simulink model "Reforce_Experiment_FCS"  (R2021a)
settings: Solver=FixedStepDiscrete  StartTime=0.0  StopTime=Inf  FixedStep=Ts  RelTol=1e-3
PostLoadFcn:
  | , if any(exist('dsrtsu_mdlpostloadfcn', 'file') ~= 0), dsrtsu_mdlpostloadfcn('Execute', bdroot); end,
InitFcn:
  | , if any(exist('rtifpga_mdlclblib', 'file') ~= 0), rtifpga_mdlclblib('Init', bdroot); end,
model workspace (MAT data in the model file):
  FPGA_Control_Scheme_1_Buffer_1_1_1_write : Simulink.Signal (value not decoded)
  FPGA_Control_Scheme_1_Buffer_2_1_1_write : Simulink.Signal (value not decoded)
  FPGA_Control_Scheme_1_Register_1_1_1_write : Simulink.Signal (value not decoded)
  FPGA_Control_Scheme_1_Register_2_1_1_write : Simulink.Signal (value not decoded)
values from neighbouring files (symbols this model uses):
  abc2alphabeta0 = [      2/3      -1/3       -1/3 ... (first row only)    [Reforce_Init.m]
  alphabeta02abc = [  1          0 1/sqrt(2) ... (first row only)    [Reforce_Init.m]
  torque_ref_sample_lower = -torque_ref_sample_upper    (= -6.5)    [Reforce_Init.m]
  torque_ref_sample_upper = 6.5    [Reforce_Init.m]
  Ts = 50e-6    (= 5e-05)    [Reforce_Init.m]
undefined symbols (not defined in the file or in its folder): controller, gcbh, init_layer_0, init_layer_1, init_layer_2, init_layer_3, init_layer_4, init_layer_5, init_layer_6, init_layer_7, init_layer_8, init_layer_9, inverter, load, motor, PLL, rtimp_mpsetup_gui, sensor
libraries: simulink x14, rtiproclib x13, rti1202lib_adc_class1 x8, rti1202lib_dio_class1 x4, dspfdesign x4, rtiemclib x2, rti1202lib_dac_class1 x1, embmathops x1, rti1202lib_base x1, rtitasklib x1, dsextras x1, simulink_extras x1
(part 5 of 5)

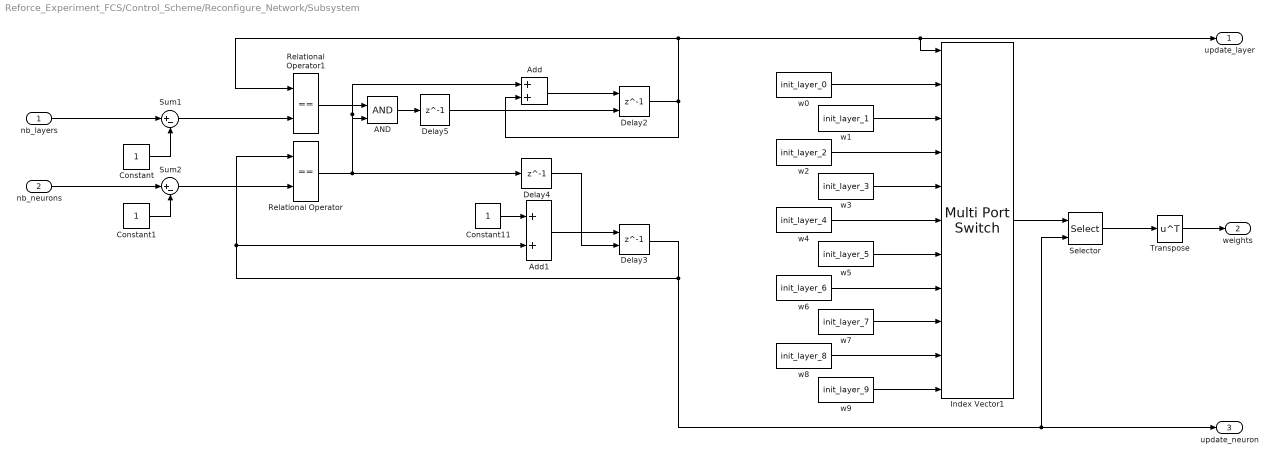
== system Reforce_Experiment_FCS/Control_Scheme/Reconfigure_Network/Subsystem ==
  nb_layers : Inport
  nb_neurons : Inport  Port=2
  AND : Logic  IconShape=distinctive  AllPortsSameDT=off  OutDataTypeStr=boolean
  Add : Sum
  Add1 : Sum
  Constant : Constant
  Constant1 : Constant
  Constant11 : Constant
  Delay2 : Delay  DelayLength=1  ExternalReset=Rising
      settings: InputPortMap=u0,r5
  Delay3 : Delay  DelayLength=1  ExternalReset=Level hold
      settings: InputPortMap=u0,r5
  Delay4 : Delay  DelayLength=1
  Delay5 : Delay  DelayLength=1
  Index Vector1 : MultiPortSwitch  DataPortOrder=Zero-based contiguous  Inputs=10  zeroidx=on
  Relational Operator : RelationalOperator  Operator===  OutDataTypeStr=boolean  RndMeth=Simplest
  Relational Operator1 : RelationalOperator  Operator===  OutDataTypeStr=boolean  RndMeth=Simplest
  Selector : Selector  NumberOfDimensions=2  IndexMode=Zero-based  InputPortWidth=2  IndexOptions=Index vector (port),Select all  Indices=[1 3],1  OutputSizes=1,1
  Sum1 : Sum  Inputs=|+-
  Sum2 : Sum  Inputs=|+-
  Transpose : Math  Operator=transpose  SaturateOnIntegerOverflow=on
  w0 : Constant  Value=init_layer_0
  w1 : Constant  Value=init_layer_1
  w2 : Constant  Value=init_layer_2
  w3 : Constant  Value=init_layer_3
  w4 : Constant  Value=init_layer_4
  w5 : Constant  Value=init_layer_5
  w6 : Constant  Value=init_layer_6
  w7 : Constant  Value=init_layer_7
  w8 : Constant  Value=init_layer_8
  w9 : Constant  Value=init_layer_9
  update_layer : Outport
  weights : Outport  Port=2
  update_neuron : Outport  Port=3
  wires:
  Delay3/1 -> Add1/2, Relational Operator/1, update_neuron/1, Selector/2
  Relational Operator/1 -> AND/2, Add/1, Delay4/1
  Add1/1 -> Delay3/1
  AND/1 -> Delay5/1
  Selector/1 -> Transpose/1
  Index Vector1/1 -> Selector/1
  Delay5/1 -> Delay2/2
  Delay2/1 -> Relational Operator1/1, update_layer/1, Index Vector1/1, Add/2
  Sum1/1 -> Relational Operator1/2
  Constant/1 -> Sum1/2
  Delay4/1 -> Delay3/2
  Add/1 -> Delay2/1
  Constant11/1 -> Add1/1
  nb_neurons/1 -> Sum2/1
  Relational Operator1/1 -> AND/1
  Sum2/1 -> Relational Operator/2
  Constant1/1 -> Sum2/2
  Transpose/1 -> weights/1
  nb_layers/1 -> Sum1/1
  w0/1 -> Index Vector1/2
  w1/1 -> Index Vector1/3
  w2/1 -> Index Vector1/4
  w3/1 -> Index Vector1/5
  w4/1 -> Index Vector1/6
  w5/1 -> Index Vector1/7
  w6/1 -> Index Vector1/8
  w7/1 -> Index Vector1/9
  w8/1 -> Index Vector1/10
  w9/1 -> Index Vector1/11

== system Reforce_Experiment_FCS/Measurement/PLL/PLL ==
  note: %% PLL
      | PLL.fn  =  50;           % [Hz] closed-loop nominal frequency of PLL
      | PLL.d   =  1;            % [] closed-loop damping factor of PLL
      | PLL.Ki_Ta = (2*pi*PLL.fn)^2;    % [1/s^2] integral gain of PLL controller
      | PLL.Kp = 2*PLL.d*2*pi*PLL.fn;   % [1/s] proportional gain of PLL controller
  note: PLL advanced entfernt
  Ts : Inport
  phi_el_cs : Inport  Port=2
  Integrator : Subsystem
  Memory : Memory  InitialCondition=[1 0]  InheritSampleTime=on  LinearizeAsDelay=on
  PI-Regler : Subsystem
  phase discriminator : Subsystem
  rad2cs : Subsystem
  Omega_el : Outport
  wires:
  Ts/1 -> PI-Regler/1(Ts), Integrator/1(Ts [s])
  Memory/1 -> phase discriminator/2(phi_e[cs])  "phi [cs]"
  rad2cs/1(phi_p[cs]) -> Memory/1  "phi_p [cs]"
  phase discriminator/1(dphi) -> PI-Regler/2(dphi)
  Integrator/1(phi [rad]) -> rad2cs/1(phi)
  PI-Regler/2(omega (KP)) -> Integrator/2(omega [rad/s])
  PI-Regler/1(omega) -> Omega_el/1  "sig_omega"
  phi_el_cs/1 -> phase discriminator/1(phi_x[cs])

== system Reforce_Experiment_FCS/Measurement/PLL/angle modulo ==
  angle_rad : Inport
  Complex to Magnitude-Angle : ComplexToMagnitudeAngle  Output=Angle
  Magnitude-Angle to Complex : MagnitudeAngleToComplex  Input=Angle  ConstantPart=1
  "angle_[-pi, pi]" : Outport
  wires:
  Magnitude-Angle to Complex/1 -> Complex to Magnitude-Angle/1
  angle_rad/1 -> Magnitude-Angle to Complex/1
  Complex to Magnitude-Angle/1 -> "angle_[-pi, pi]"/1

== system Reforce_Experiment_FCS/Measurement/abc2dq/alphabeta02dq ==
  alphabeta0 : Inport
  epsilon : Inport  Port=2
  Cos : Trigonometry  Operator=cos  NumberOfDataPoints=64
  Demux : Demux  Outputs=3
  Gain1 : Gain  Gain=-1
  Gain2 : Gain  Gain=-1
  Mux : Mux  Inputs=2
  Product{,1..3} (4 alike) : Product
  Sin : Trigonometry  NumberOfDataPoints=64
  Sum : Sum  Inputs=|++
  Sum1 : Sum  Inputs=|++
  Terminator : Terminator
  dq : Outport
  wires:
  epsilon/1 -> Gain2/1
  alphabeta0/1 -> Demux/1
  Demux/3 -> Terminator/1
  Sum/1 -> Mux/1
  Sum1/1 -> Mux/2
  Mux/1 -> dq/1
  Demux/1 -> Product1/1, Product2/1
  Cos/1 -> Product1/2, Product3/2
  Product1/1 -> Sum/1
  Demux/2 -> Product3/1, Product/1
  Gain1/1 -> Product/2
  Product/1 -> Sum/2
  Product2/1 -> Sum1/1
  Sin/1 -> Gain1/1, Product2/2
  Product3/1 -> Sum1/2
  Gain2/1 -> Sin/1, Cos/1

== system Reforce_Experiment_FCS/RTI Data/RTI Data Store/RTI Data Store ==
  RTI Data Store : Subsystem  mask(RTI_DATA_STORE){}
      mask help:
      | RTI Data Store Block. This block is used by RTI to store internal model dependent data. Deleting this block will result in data loss.
      |
      | NEVER DELETE, COPY, OR MODIFY THIS BLOCK!
      mask Help:
      | RTI Data Store Block. This block is used by RTI to store internal model dependent data. Deleting this block will result in data loss.
      | 
      | NEVER DELETE, COPY, OR MODIFY THIS BLOCK!
      mask Display: text(0.5, 0.5, ' ', 'HorizontalAlignment', 'center');

== system Reforce_Experiment_FCS/Control_Scheme/DQ_DTC/Action_Processing/argmax ==
  Q_values : Inport
  Add : Sum  Inputs=+-
  Compare To Zero : simulink/Logic and Bit Operations/Compare To Zero  relop===  OutDataTypeStr=boolean
  Find Nonzero Elements : Find  NumberOfInputDimensions=3  IndexMode=Zero-based
  Max : MinMax  Function=max
  Min : MinMax
  Rate Transition : RateTransition  Commented=on
  argmax_Q : Outport
  wires:
  Q_values/1 -> Add/1, Max/1
  Max/1 -> Add/2
  Add/1 -> Compare To Zero/1
  Find Nonzero Elements/1 -> Min/1
  Min/1 -> argmax_Q/1
  Compare To Zero/1 -> Find Nonzero Elements/1

== system Reforce_Experiment_FCS/Control_Scheme/DQ_DTC/Featurizer/DC_link_scaling ==
  u_DC : Inport
  Add : Sum  Inputs=+-
  Add1 : Sum  Inputs=-+
  Add2 : Sum  Inputs=+-
  Constant : Constant  Value=controller.DQDTC.u_DC_max
  Constant1 : Constant  Value=controller.DQDTC.u_DC_min
  Constant2 : Constant
  Divide : Product  Inputs=*/
  Gain : Gain  Gain=2
  u_DC_norm : Outport
  wires:
  u_DC/1 -> Add/1
  Constant1/1 -> Add/2, Add1/1
  Add/1 -> Divide/1
  Constant/1 -> Add1/2
  Add1/1 -> Divide/2
  Divide/1 -> Gain/1
  Constant2/1 -> Add2/2
  Add2/1 -> u_DC_norm/1
  Gain/1 -> Add2/1

== system Reforce_Experiment_FCS/Control_Scheme/DQ_DTC/Featurizer/stator_current_scaling ==
  i_dq_norm : Inport
  Constant : Constant
  Demux : Demux  Outputs=2
  Gain1 : Gain  Gain=2
  Sqrt : Sqrt  SaturateOnIntegerOverflow=on
  Square : Math  Operator=square  SaturateOnIntegerOverflow=on
  Square1 : Math  Operator=square  SaturateOnIntegerOverflow=on
  Sum : Sum  Inputs=|++
  Sum1 : Sum  Inputs=|+-
  i_s_norm : Outport
  wires:
  Constant/1 -> Sum1/2
  Gain1/1 -> Sum1/1
  Square/1 -> Sum/1
  Sqrt/1 -> Gain1/1
  i_dq_norm/1 -> Demux/1
  Demux/2 -> Square1/1
  Sum/1 -> Sqrt/1
  Demux/1 -> Square/1
  Square1/1 -> Sum/2
  Sum1/1 -> i_s_norm/1

== system Reforce_Experiment_FCS/Control_Scheme/DQ_DTC/Identification_and_Safeguard/A_d_static ==
  w_me : Inport
  Constant : Constant  Value=-1/motor.param.tau_d
  Constant1 : Constant  Value=-1/motor.param.tau_q
  Constant2 : Constant  Value=eye(2)
  Gain : Gain  Gain=-motor.param.L_d / motor.param.L_q
  Gain1 : Gain  Gain=motor.param.L_q / motor.param.L_d
  Gain2 : Gain  Gain=motor.param.p
  Gain3 : Gain  Gain=Ts
  Mux : Mux
  Plus : Sum
  Reshape1 : Reshape  OutputDimensionality=Customize  OutputDimensions=[2,2]
  A_d : Outport
  wires:
  Mux/1 -> Reshape1/1
  Constant/1 -> Mux/1
  Constant1/1 -> Mux/4
  Gain/1 -> Mux/2
  w_me/1 -> Gain2/1
  Gain2/1 -> Gain1/1, Gain/1
  Gain1/1 -> Mux/3
  Reshape1/1 -> Gain3/1
  Gain3/1 -> Plus/2
  Constant2/1 -> Plus/1
  Plus/1 -> A_d/1

== system Reforce_Experiment_FCS/Control_Scheme/DQ_DTC/Identification_and_Safeguard/Brosch RLS ==
  reset : Inport
  i_dq : Inport  Port=2
  u_dq : Inport  Port=3
  Routing : Subsystem
  i_d_RLS : Subsystem
  lambda : Constant  Value=controller.RLS.lambda
  A : Outport
  B : Outport  Port=2
  E : Outport  Port=3
  wires:
  Routing/3(E) -> E/1
  u_dq/1 -> i_d_RLS/3(u_dq)
  i_dq/1 -> i_d_RLS/2(i_dq)
  Routing/2(B) -> B/1
  i_d_RLS/1(theta_d_k) -> Routing/1(theta_d)
  Routing/1(A) -> A/1
  lambda/1 -> i_d_RLS/4(lambda)
  reset/1 -> i_d_RLS/1(reset)
  i_d_RLS/2(theta_q_k) -> Routing/2(theta_q)

== system Reforce_Experiment_FCS/Control_Scheme/DQ_DTC/Identification_and_Safeguard/DeadTimeCompensationPredictor ==
  A : Inport
  B : Inport  Port=2
  E : Inport  Port=3
  i_dq : Inport  Port=4
  u_dq : Inport  Port=5
  Add : Sum  Inputs=3
  Matrix Multiply : Product  Multiplication=Matrix(*)
  Matrix Multiply1 : Product  Multiplication=Matrix(*)
  i_dq[k+1] : Outport
  wires:
  i_dq/1 -> Matrix Multiply/2
  Add/1 -> i_dq[k+1]/1
  B/1 -> Matrix Multiply1/1
  Matrix Multiply/1 -> Add/1
  A/1 -> Matrix Multiply/1
  u_dq/1 -> Matrix Multiply1/2
  Matrix Multiply1/1 -> Add/2
  E/1 -> Add/3

== system Reforce_Experiment_FCS/Control_Scheme/DQ_DTC/Identification_and_Safeguard/E_d_static ==
  w_me : Inport
  Constant : Constant  Value=0
  Gain : Gain  Gain=-motor.param.p*motor.param.psi_p/motor.param.L_q
  Gain1 : Gain  Gain=Ts
  Mux : Mux  Inputs=2
  E_d : Outport
  wires:
  Mux/1 -> E_d/1
  Constant/1 -> Mux/1
  w_me/1 -> Gain/1
  Gain/1 -> Gain1/1
  Gain1/1 -> Mux/2

== system Reforce_Experiment_FCS/Control_Scheme/DQ_DTC/Identification_and_Safeguard/Horizon1Predictor ==
  A : Inport
  B : Inport  Port=2
  E : Inport  Port=3
  lastControlSignal : Inport  Port=4
  u_DC : Inport  Port=5
  i_dq[k+1] : Inport  Port=6
  i_abc[k+1] : Inport  Port=7
  epsilon : Inport  Port=8
  T_interlock : Inport  Port=9
  i_threshold : Inport  Port=10
  Constant : Constant  Value=inverter.mapping
  Constant1 : Constant  Value=eye(2)
  Constant3 : Constant  Value=[0 0]
  For Each Subsystem : Subsystem  TreatAsAtomicUnit=on
  Matrix Multiply : Product  Multiplication=Matrix(*)
  Matrix Multiply2 : Product  Inputs=/  Multiplication=Matrix(*)
  Plus : Sum
  Plus1 : Sum  Inputs=+-
  all_i_dq[k+2] : Outport
  all_u_EMF[k+2] : Outport  Port=2
  wires:
  E/1 -> Plus/1, For Each Subsystem/1(E)
  A/1 -> Matrix Multiply/1, Plus1/2
  Matrix Multiply/1 -> Plus/2
  Constant/1 -> For Each Subsystem/6(nextControlSignal)
  Constant1/1 -> Plus1/1
  i_threshold/1 -> For Each Subsystem/12(i_threshold)
  T_interlock/1 -> For Each Subsystem/11(T_interlock)
  i_abc[k+1]/1 -> For Each Subsystem/9(i_abc)
  u_DC/1 -> For Each Subsystem/8(u_DC)
  Matrix Multiply2/1 -> For Each Subsystem/5(B_inv)
  B/1 -> Matrix Multiply2/1, For Each Subsystem/4(B)
  Plus1/1 -> For Each Subsystem/2(I_minus_A)
  Plus/1 -> For Each Subsystem/3(Ai_plus_E)
  For Each Subsystem/2(u_dq[k+2]) -> all_u_EMF[k+2]/1
  For Each Subsystem/1(i_dq[k+2]) -> all_i_dq[k+2]/1
  lastControlSignal/1 -> For Each Subsystem/7(lastControlSignal)
  Constant3/1 -> Matrix Multiply/2
  epsilon/1 -> For Each Subsystem/10(epsilon)

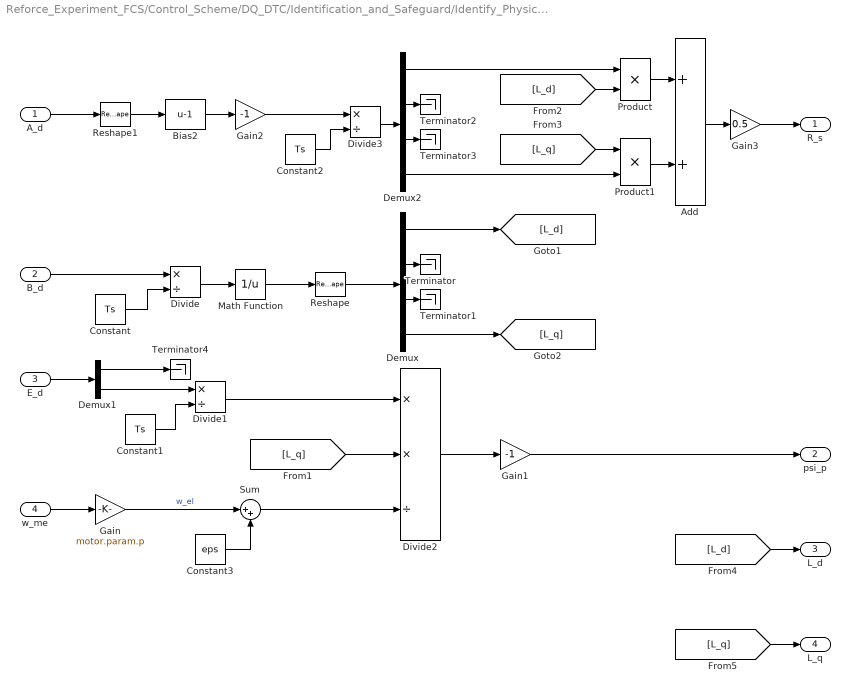
== system Reforce_Experiment_FCS/Control_Scheme/DQ_DTC/Identification_and_Safeguard/Identify_Physical_Parameters ==
  A_d : Inport
  B_d : Inport  Port=2
  E_d : Inport  Port=3
  w_me : Inport  Port=4
  Add : Sum
  Bias2 : Bias  Bias=-1
  Constant : Constant  Value=Ts
  Constant1 : Constant  Value=Ts
  Constant2 : Constant  Value=Ts
  Constant3 : Constant  Value=eps
  Demux : Demux
  Demux1 : Demux  Outputs=2
  Demux2 : Demux
  Divide : Product  Inputs=*/
  Divide1 : Product  Inputs=*/
  Divide2 : Product  Inputs=**/
  Divide3 : Product  Inputs=*/
  Gain : Gain  Gain=motor.param.p
  Gain1 : Gain  Gain=-1
  Gain2 : Gain  Gain=-1
  Gain3 : Gain  Gain=0.5
  Math Function : Math  Operator=reciprocal  SaturateOnIntegerOverflow=on
  Product : Product
  Product1 : Product
  Reshape : Reshape
  Reshape1 : Reshape
  Sum : Sum  Inputs=|++
  Terminator{,1..4} (5 alike) : Terminator
  R_s : Outport
  psi_p : Outport  Port=2
  L_d : Outport  Port=3
  L_q : Outport  Port=4
  wires:
  B_d/1 -> Divide/1
  Constant/1 -> Divide/2
  w_me/1 -> Gain/1
  Constant1/1 -> Divide1/2
  Divide1/1 -> Divide2/1
  Demux/1 -> [L_d]
  Reshape/1 -> Demux/1
  Demux/4 -> [L_q]
  Math Function/1 -> Reshape/1
  Demux/2 -> Terminator/1
  Demux/3 -> Terminator1/1
  Divide/1 -> Math Function/1
  [L_q] -> Divide2/2
  Divide2/1 -> Gain1/1
  Gain1/1 -> psi_p/1
  Reshape1/1 -> Bias2/1
  Demux2/3 -> Terminator3/1
  Demux2/2 -> Terminator2/1
  Bias2/1 -> Gain2/1
  A_d/1 -> Reshape1/1
  Constant2/1 -> Divide3/2
  Divide3/1 -> Demux2/1
  Gain2/1 -> Divide3/1
  Product/1 -> Add/1
  Product1/1 -> Add/2
  Add/1 -> Gain3/1
  Gain3/1 -> R_s/1
  Demux2/1 -> Product/1
  Demux2/4 -> Product1/2
  [L_q] -> Product1/1
  [L_d] -> Product/2
  [L_q] -> L_q/1
  [L_d] -> L_d/1
  Gain/1 -> Sum/1  "w_el"
  Sum/1 -> Divide2/3
  Constant3/1 -> Sum/2
  E_d/1 -> Demux1/1
  Demux1/2 -> Divide1/1
  Demux1/1 -> Terminator4/1

== system Reforce_Experiment_FCS/Control_Scheme/DQ_DTC/Identification_and_Safeguard/Safeguard ==
  i_dq : Inport
  u_dq : Inport  Port=2
  u_DC : Inport  Port=3
  Constant : Constant  Value=1:16
  Constant8 : Constant  Value=0:7
  For Each Subsystem : Subsystem  TreatAsAtomicUnit=on
  a_allowed : Outport
  all_i_s_feat : Outport  Port=2
  wires:
  u_dq/1 -> For Each Subsystem/2(u_dq)
  u_DC/1 -> For Each Subsystem/3(u_DC)
  For Each Subsystem/1(violation) -> a_allowed/1
  Constant8/1 -> For Each Subsystem/4(switch_state_index)
  For Each Subsystem/2(i_s_norm) -> all_i_s_feat/1
  Constant/1 -> For Each Subsystem/1(i_dq)

== system Reforce_Experiment_FCS/Control_Scheme/DQ_DTC/Identification_and_Safeguard/dq2abc ==
  dq : Inport
  epsilon : Inport  Port=2
  Gain1 : Gain  Gain=alphabeta02abc  Multiplication=Matrix(K*u)
  alphabeta02dq : Subsystem
  abc : Outport
  wires:
  epsilon/1 -> alphabeta02dq/2(epsilon)
  alphabeta02dq/1(alphabeta0) -> Gain1/1
  Gain1/1 -> abc/1
  dq/1 -> alphabeta02dq/1(dq)

== system Reforce_Experiment_FCS/Control_Scheme/DQ_DTC/Reward function/Zone A ==
  i_s : Inport
  Action Port : ActionPort  ActionPortLabel=else
  Add : Sum  Inputs=+-
  Constant : Constant
  Constant2 : Constant  Value=(controller.DQDTC.reward_interval)/2
  Constant3 : Constant  Value=0
  Gain1 : Gain  Gain=controller.DQDTC.reward_interval / 2
  Sum : Sum  Inputs=|++
  reward : Outport
  done : Outport  Port=2
  wires:
  Constant/1 -> Add/1
  i_s/1 -> Add/2
  Add/1 -> Gain1/1
  Gain1/1 -> Sum/1
  Sum/1 -> reward/1
  Constant2/1 -> Sum/2
  Constant3/1 -> done/1

== system Reforce_Experiment_FCS/Control_Scheme/DQ_DTC/Reward function/Zone B ==
  e_T_norm : Inport
  Action Port : ActionPort  ActionPortLabel=elseif( u3 > u5)
  Add1 : Sum  Inputs=+-
  Constant1 : Constant
  Constant3 : Constant  Value=0
  Gain : Gain  Gain=1/2
  Gain1 : Gain  Gain=controller.DQDTC.reward_interval / 2
  reward : Outport
  done : Outport  Port=2
  wires:
  Constant3/1 -> done/1
  Add1/1 -> Gain1/1
  Constant1/1 -> Add1/1
  e_T_norm/1 -> Gain/1
  Gain1/1 -> reward/1
  Gain/1 -> Add1/2

== system Reforce_Experiment_FCS/Control_Scheme/DQ_DTC/Reward function/Zone BS ==
  Action Port : ActionPort  ActionPortLabel=elseif( u7>0)
  Constant1 : Constant  Value=0
  Constant3 : Constant  Value=0
  reward : Outport
  done : Outport  Port=2
  wires:
  Constant3/1 -> done/1
  Constant1/1 -> reward/1

== system Reforce_Experiment_FCS/Control_Scheme/DQ_DTC/Reward function/Zone C ==
  i_d_norm : Inport
  Action Port : ActionPort  ActionPortLabel=elseif( u1 >= u6)
  Add : Sum  Inputs=+-
  Add1 : Sum  Inputs=+-
  Constant : Constant  Value=controller.DQDTC.i_d_plus_norm
  Constant1 : Constant
  Constant2 : Constant  Value=(controller.DQDTC.reward_interval)/2
  Constant3 : Constant  Value=0
  Gain : Gain  Gain=1/(controller.DQDTC.i_nominal_norm-controller.DQDTC.i_d_plus_norm)
  Gain1 : Gain  Gain=controller.DQDTC.reward_interval / 2
  Sum : Sum  Inputs=|+-
  reward : Outport
  done : Outport  Port=2
  wires:
  Constant3/1 -> done/1
  Add1/1 -> Gain1/1
  i_d_norm/1 -> Add/1
  Constant/1 -> Add/2
  Constant1/1 -> Add1/1
  Add/1 -> Gain/1
  Constant2/1 -> Sum/2
  Sum/1 -> reward/1
  Gain/1 -> Add1/2
  Gain1/1 -> Sum/1

== system Reforce_Experiment_FCS/Control_Scheme/DQ_DTC/Reward function/Zone D ==
  i_s_norm : Inport
  Action Port : ActionPort  ActionPortLabel=elseif(u2 >= u4)
  Add : Sum  Inputs=+-
  Add1 : Sum  Inputs=+-
  Constant : Constant  Value=controller.DQDTC.i_nominal_norm
  Constant1 : Constant
  Constant2 : Constant  Value=controller.DQDTC.reward_interval
  Constant3 : Constant  Value=0
  Gain : Gain  Gain=1/(1-controller.DQDTC.i_nominal_norm)
  Gain1 : Gain  Gain=controller.DQDTC.reward_interval / 2
  Sum : Sum  Inputs=|+-
  reward : Outport
  done : Outport  Port=2
  wires:
  i_s_norm/1 -> Add/1
  Constant/1 -> Add/2
  Add/1 -> Gain/1
  Constant1/1 -> Add1/1
  Gain/1 -> Add1/2
  Add1/1 -> Gain1/1
  Gain1/1 -> Sum/1
  Sum/1 -> reward/1
  Constant2/1 -> Sum/2
  Constant3/1 -> done/1

== system Reforce_Experiment_FCS/Control_Scheme/DQ_DTC/Reward function/Zone DS ==
  Action Port : ActionPort  ActionPortLabel=elseif( (u7 > 0) & (u8 > u4))
  Constant2 : Constant  Value=-(controller.DQDTC.reward_interval)/2
  Constant3 : Constant  Value=0
  reward : Outport
  done : Outport  Port=2
  wires:
  Constant3/1 -> done/1
  Constant2/1 -> reward/1

== system Reforce_Experiment_FCS/Control_Scheme/DQ_DTC/Reward function/Zone E ==
  Action Port : ActionPort  ActionPortLabel=if(u2 >= 1)
  Constant : Constant  Value=-1
  Constant1 : Constant
  reward : Outport
  done : Outport  Port=2
  wires:
  Constant/1 -> reward/1
  Constant1/1 -> done/1

== system Reforce_Experiment_FCS/Control_Scheme/DQ_DTC/Reward function/Zone ES ==
  Action Port : ActionPort  ActionPortLabel=elseif(u8>=1)
  Constant1 : Constant  Value=0
  Constant2 : Constant  Value=-controller.DQDTC.reward_interval
  reward : Outport
  done : Outport  Port=2
  wires:
  Constant2/1 -> reward/1
  Constant1/1 -> done/1

== system Reforce_Experiment_FCS/Control_Scheme/DQ_DTC/abc2dq1/alphabeta02dq ==
  alphabeta0 : Inport
  epsilon : Inport  Port=2
  Cos : Trigonometry  Operator=cos  NumberOfDataPoints=64
  Demux : Demux  Outputs=3
  Gain1 : Gain  Gain=-1
  Gain2 : Gain  Gain=-1
  Mux : Mux  Inputs=2
  Product{,1..3} (4 alike) : Product
  Sin : Trigonometry  NumberOfDataPoints=64
  Sum : Sum  Inputs=|++
  Sum1 : Sum  Inputs=|++
  Terminator : Terminator
  dq : Outport
  wires:
  Gain2/1 -> Cos/1, Sin/1
  Product3/1 -> Sum1/2
  Sin/1 -> Product2/2, Gain1/1
  Product2/1 -> Sum1/1
  Product/1 -> Sum/2
  Gain1/1 -> Product/2
  Demux/2 -> Product/1, Product3/1
  Product1/1 -> Sum/1
  Cos/1 -> Product3/2, Product1/2
  Demux/1 -> Product2/1, Product1/1
  Mux/1 -> dq/1
  Sum1/1 -> Mux/2
  Sum/1 -> Mux/1
  Demux/3 -> Terminator/1
  alphabeta0/1 -> Demux/1
  epsilon/1 -> Gain2/1

== system Reforce_Experiment_FCS/Measurement/PLL/PLL/Integrator ==
  Ts [s] : Inport
  omega [rad/s] : Inport  Port=2
  Memory : Memory  InheritSampleTime=on  LinearizeAsDelay=on
  Product5 : Product  Inputs=**  InputSameDT=on  RndMeth=Zero  SaturateOnIntegerOverflow=on  OutDataTypeStr=Inherit: Same as first input
  phi_me : Sum  InputSameDT=on  SaturateOnIntegerOverflow=on  OutDataTypeStr=Inherit: Same as first input
  phi [rad] : Outport
  wires:
  Product5/1 -> phi_me/1
  phi_me/1 -> phi [rad]/1, Memory/1  "phi_me_p"
  Memory/1 -> phi_me/2
  Ts [s]/1 -> Product5/1
  omega [rad/s]/1 -> Product5/2

== system Reforce_Experiment_FCS/Measurement/PLL/PLL/PI-Regler ==
  Ts : Inport
  dphi : Inport  Port=2
  Memory : Memory  InheritSampleTime=on  LinearizeAsDelay=on
  PLL_Ki : Gain  Gain=PLL.Ki_Ta  SaturateOnIntegerOverflow=on  OutDataTypeStr=Inherit: Same as input  ParamDataTypeStr=Inherit: Same as input
  PLL_Kp : Gain  Gain=PLL.Kp  SaturateOnIntegerOverflow=on  OutDataTypeStr=Inherit: Same as input  ParamDataTypeStr=Inherit: Same as input
  Product6 : Product  Inputs=**  InputSameDT=on  RndMeth=Zero  SaturateOnIntegerOverflow=on  OutDataTypeStr=Inherit: Same as first input
  Sum2 : Sum  InputSameDT=on  SaturateOnIntegerOverflow=on  OutDataTypeStr=Inherit: Same as first input
  Sum_om : Sum  InputSameDT=on  SaturateOnIntegerOverflow=on  OutDataTypeStr=Inherit: Same as first input
  omega : Outport
  omega (KP) : Outport  Port=2
  wires:
  Product6/1 -> Sum2/1
  dphi/1 -> PLL_Ki/1, PLL_Kp/1
  PLL_Ki/1 -> Product6/2
  Sum2/1 -> Memory/1
  Memory/1 -> Sum_om/1, omega/1, Sum2/2  "omega"
  PLL_Kp/1 -> Sum_om/2
  Sum_om/1 -> omega (KP)/1  "om"
  Ts/1 -> Product6/1

== system Reforce_Experiment_FCS/Measurement/PLL/PLL/phase discriminator ==
  phi_x[cs] : Inport  PortDimensions=2
  phi_e[cs] : Inport  Port=2  PortDimensions=2
  Demux : Demux  Outputs=2
      settings: DisplayOption=none
  Demux1 : Demux  Outputs=2
      settings: DisplayOption=none
  Product : Product  Inputs=**  InputSameDT=on  RndMeth=Zero  SaturateOnIntegerOverflow=on  OutDataTypeStr=Inherit: Same as first input
  Product1 : Product  Inputs=**  InputSameDT=on  RndMeth=Zero  SaturateOnIntegerOverflow=on  OutDataTypeStr=Inherit: Same as first input
  dphi1 : Sum  Inputs=-+  InputSameDT=on  SaturateOnIntegerOverflow=on  OutDataTypeStr=Inherit: Same as first input
  dphi : Outport
  wires:
  dphi1/1 -> dphi/1
  phi_e[cs]/1 -> Demux/1
  Demux1/2 -> Product1/1
  Demux/1 -> Product1/2
  Demux/2 -> Product/2
  Demux1/1 -> Product/1
  Product1/1 -> dphi1/2
  Product/1 -> dphi1/1
  phi_x[cs]/1 -> Demux1/1

== system Reforce_Experiment_FCS/Measurement/PLL/PLL/rad2cs ==
  phi : Inport  PortDimensions=1
  Mux4 : Mux  Inputs=2
  angle modulo : Subsystem
  cos : Trigonometry  Operator=cos  NumberOfDataPoints=64
  sin : Trigonometry  NumberOfDataPoints=64
  phi_p[cs] : Outport
  wires:
  angle modulo/1("angle_[-pi, pi]") -> cos/1, sin/1
  phi/1 -> angle modulo/1(angle_rad)
  cos/1 -> Mux4/1
  sin/1 -> Mux4/2
  Mux4/1 -> phi_p[cs]/1

== system Reforce_Experiment_FCS/RTI Data/RTI Data Store/RTI Data Store/RTI Data Store ==
  RTI Data Store : Subsystem  mask(RTI_DATA_STORE){}
      mask help:
      | RTI Data Store Block. This block is used by RTI to store internal model dependent data. Deleting this block will result in data loss.
      |
      | NEVER DELETE, COPY, OR MODIFY THIS BLOCK!
      mask Help:
      | RTI Data Store Block. This block is used by RTI to store internal model dependent data. Deleting this block will result in data loss.
      | 
      | NEVER DELETE, COPY, OR MODIFY THIS BLOCK!
      mask Display: text(0.5, 0.5, ' ', 'HorizontalAlignment', 'center');

== system Reforce_Experiment_FCS/Control_Scheme/DQ_DTC/Identification_and_Safeguard/Brosch RLS/Routing ==
  theta_d : Inport
  theta_q : Inport  Port=2
  Demux : Demux  Outputs=5
  Demux1 : Demux  Outputs=5
  Mux : Mux
  Mux1 : Mux
  Mux2 : Mux  Inputs=2
  Reshape1 : Reshape  OutputDimensionality=Customize  OutputDimensions=[2,2]
  Reshape2 : Reshape  OutputDimensionality=Customize  OutputDimensions=[2,2]
  A : Outport
  B : Outport  Port=2
  E : Outport  Port=3
  wires:
  Demux/3 -> Mux1/1
  Demux1/1 -> Mux/2
  Demux1/5 -> Mux2/2
  Demux1/2 -> Mux/4
  Mux2/1 -> E/1
  Demux/1 -> Mux/1
  Demux/4 -> Mux1/3
  Demux/2 -> Mux/3
  Demux1/4 -> Mux1/4
  Demux1/3 -> Mux1/2
  Mux/1 -> Reshape1/1
  Demux/5 -> Mux2/1
  Mux1/1 -> Reshape2/1
  theta_d/1 -> Demux/1
  Reshape2/1 -> B/1
  theta_q/1 -> Demux1/1
  Reshape1/1 -> A/1

== system Reforce_Experiment_FCS/Control_Scheme/DQ_DTC/Identification_and_Safeguard/Brosch RLS/i_d_RLS ==
  reset : Inport
  i_dq : Inport  Port=2
  u_dq : Inport  Port=3
  lambda : Inport  Port=4
  Constant : Constant
  Delay : Delay  DelayLength=1  InitialCondition=controller.RLS.xi_0
  Mux : Mux  Inputs=3
  RLS : Subsystem
  Subsystem : Subsystem
  Subsystem2 : Subsystem
  theta_d_k : Outport
  theta_q_k : Outport  Port=2
  wires:
  Constant/1 -> Mux/3
  i_dq/1 -> RLS/4(psi_k), Mux/1
  Mux/1 -> Delay/1
  u_dq/1 -> Mux/2
  Delay/1 -> RLS/2(xi_k), Subsystem/1(xi_k), Subsystem2/2(xi_k)
  Subsystem2/1(P_k-1) -> Subsystem/2(P_k-1)
  reset/1 -> Subsystem2/1(reset), RLS/1(reset)
  Subsystem/1(gamma_k-1) -> RLS/3(gamma_k-1), Subsystem2/3(gamma_k-1)
  lambda/1 -> Subsystem/3(lambda), Subsystem2/4(lambda)
  RLS/2(theta_q_k1) -> theta_q_k/1
  RLS/1(theta_d_k) -> theta_d_k/1

== system Reforce_Experiment_FCS/Control_Scheme/DQ_DTC/Identification_and_Safeguard/Horizon1Predictor/For Each Subsystem ==
  E : Inport
  I_minus_A : Inport  Port=2
  Ai_plus_E : Inport  Port=3
  B : Inport  Port=4
  B_inv : Inport  Port=5
  nextControlSignal : Inport  Port=6  Partition=on  PartitionDimension=2  PartitionWidth=1  PartitionOffset=0
  lastControlSignal : Inport  Port=7
  u_DC : Inport  Port=8
  i_abc : Inport  Port=9
  epsilon : Inport  Port=10
  T_interlock : Inport  Port=11
  i_threshold : Inport  Port=12
  For Each : ForEach  DisableCoverage=on
  Predictor1 : Subsystem
  VoltageApplier1 : Subsystem
  i_dq[k+2] : Outport  ConcatenationDimension=1
  u_dq[k+2] : Outport  Port=2  ConcatenationDimension=1
  wires:
  epsilon/1 -> VoltageApplier1/5(epsilon)
  B/1 -> Predictor1/3(B)
  Predictor1/2(u_dq[k+2]) -> u_dq[k+2]/1
  nextControlSignal/1 -> VoltageApplier1/1(nextControlSignal)
  Predictor1/1(i_dq[k+2]) -> i_dq[k+2]/1
  lastControlSignal/1 -> VoltageApplier1/2(lastControlSignal)
  E/1 -> Predictor1/5(E)
  i_abc/1 -> VoltageApplier1/4(i_abc)
  B_inv/1 -> Predictor1/4(B_inv)
  u_DC/1 -> VoltageApplier1/3(u_DC)
  VoltageApplier1/1(u_dq[k+1]) -> Predictor1/6(u_dq)
  T_interlock/1 -> VoltageApplier1/6(T_interlock)
  i_threshold/1 -> VoltageApplier1/7(i_threshold)
  I_minus_A/1 -> Predictor1/2(I_minus_A)
  Ai_plus_E/1 -> Predictor1/1(Ai_plus_E)

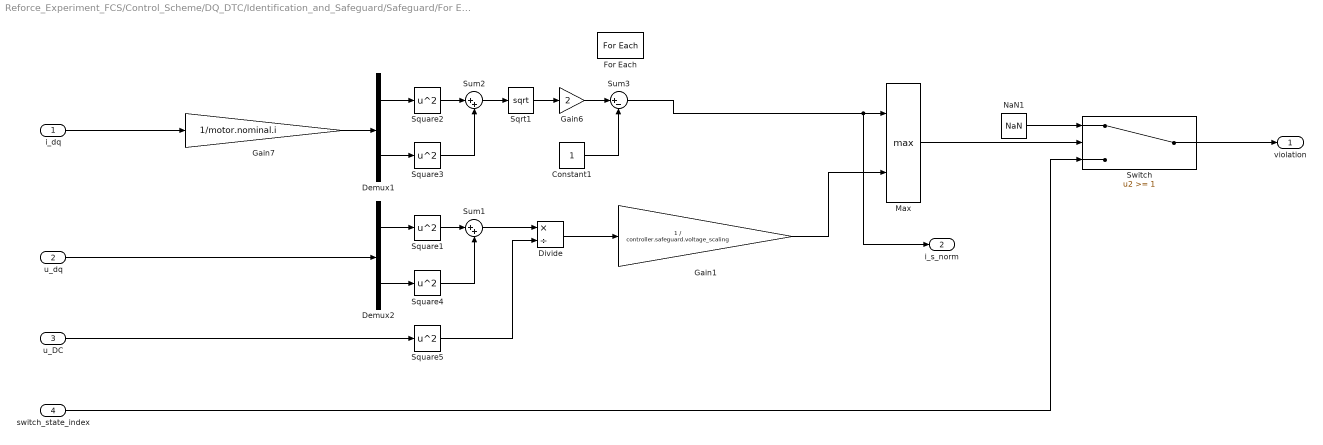
== system Reforce_Experiment_FCS/Control_Scheme/DQ_DTC/Identification_and_Safeguard/Safeguard/For Each Subsystem ==
  i_dq : Inport  Partition=on  PartitionDimension=1  PartitionWidth=2  PartitionOffset=0
  u_dq : Inport  Port=2  Partition=on  PartitionDimension=1  PartitionWidth=2  PartitionOffset=0
  u_DC : Inport  Port=3
  switch_state_index : Inport  Port=4  Partition=on  PartitionDimension=1  PartitionWidth=1  PartitionOffset=0
  Constant1 : Constant
  Demux1 : Demux  Outputs=2
  Demux2 : Demux  Outputs=2
  Divide : Product  Inputs=*/
  For Each : ForEach  DisableCoverage=on
  Gain1 : Gain  Gain=1 / controller.safeguard.voltage_scaling
  Gain6 : Gain  Gain=2
  Gain7 : Gain  Gain=1/motor.nominal.i
  Max : MinMax  Function=max  Inputs=2
  NaN1 : Constant  Value=NaN  OutDataTypeStr=Inherit: Inherit via back propagation
  Sqrt1 : Sqrt  SaturateOnIntegerOverflow=on
  Square{1..5} (5 alike) : Math  Operator=square  SaturateOnIntegerOverflow=on
  Sum1 : Sum  Inputs=|++
  Sum2 : Sum  Inputs=|++
  Sum3 : Sum  Inputs=|+-
  Switch : Switch  Threshold=1
  violation : Outport  ConcatenationDimension=1
  i_s_norm : Outport  Port=2  ConcatenationDimension=1
  wires:
  Square1/1 -> Sum1/1
  Sqrt1/1 -> Gain6/1
  Sum2/1 -> Sqrt1/1
  Square3/1 -> Sum2/2
  Constant1/1 -> Sum3/2
  Divide/1 -> Gain1/1
  Demux1/2 -> Square3/1
  Demux1/1 -> Square2/1
  Gain6/1 -> Sum3/1
  Square2/1 -> Sum2/1
  Demux2/1 -> Square1/1
  u_dq/1 -> Demux2/1
  Gain7/1 -> Demux1/1
  Square5/1 -> Divide/2
  u_DC/1 -> Square5/1
  Sum1/1 -> Divide/1
  Square4/1 -> Sum1/2
  Demux2/2 -> Square4/1
  switch_state_index/1 -> Switch/3
  NaN1/1 -> Switch/1
  Max/1 -> Switch/2
  Switch/1 -> violation/1
  Sum3/1 -> i_s_norm/1, Max/1
  i_dq/1 -> Gain7/1
  Gain1/1 -> Max/2

== system Reforce_Experiment_FCS/Control_Scheme/DQ_DTC/Identification_and_Safeguard/dq2abc/alphabeta02dq ==
  dq : Inport
  epsilon : Inport  Port=2
  Constant : Constant  Value=0
  Cos : Trigonometry  Operator=cos  NumberOfDataPoints=64
  Demux : Demux  Outputs=2
  Gain1 : Gain  Gain=-1
  Mux : Mux  Inputs=3
  Product{,1..3} (4 alike) : Product
  Sin : Trigonometry  NumberOfDataPoints=64
  Sum : Sum  Inputs=|++
  Sum1 : Sum  Inputs=|++
  alphabeta0 : Outport
  wires:
  dq/1 -> Demux/1
  Sum/1 -> Mux/1
  Sum1/1 -> Mux/2
  Mux/1 -> alphabeta0/1
  Demux/1 -> Product2/1, Product1/1
  Cos/1 -> Product1/2, Product3/2
  Product1/1 -> Sum/1
  Demux/2 -> Product3/1, Product/1
  Gain1/1 -> Product/2
  Product/1 -> Sum/2
  Product2/1 -> Sum1/1
  Sin/1 -> Gain1/1, Product2/2
  Product3/1 -> Sum1/2
  epsilon/1 -> Sin/1, Cos/1
  Constant/1 -> Mux/3

== system Reforce_Experiment_FCS/Measurement/PLL/PLL/rad2cs/angle modulo ==
  angle_rad : Inport
  Complex to Magnitude-Angle : ComplexToMagnitudeAngle  Output=Angle
  Magnitude-Angle to Complex : MagnitudeAngleToComplex  Input=Angle  ConstantPart=1
  "angle_[-pi, pi]" : Outport
  wires:
  Magnitude-Angle to Complex/1 -> Complex to Magnitude-Angle/1
  angle_rad/1 -> Magnitude-Angle to Complex/1
  Complex to Magnitude-Angle/1 -> "angle_[-pi, pi]"/1

== system Reforce_Experiment_FCS/RTI Data/RTI Data Store/RTI Data Store/RTI Data Store/RTI Data Store ==

== system Reforce_Experiment_FCS/Control_Scheme/DQ_DTC/Identification_and_Safeguard/Brosch RLS/i_d_RLS/RLS ==
  reset : Inport
  xi_k : Inport  Port=2
  gamma_k-1 : Inport  Port=3
  psi_k : Inport  Port=4
  Demux : Demux  Outputs=2
  Subsystem1 : Subsystem
  Subsystem2 : Subsystem
  theta_d_k : Outport
  theta_q_k1 : Outport  Port=2
  wires:
  gamma_k-1/1 -> Subsystem2/3(gamma_k-1), Subsystem1/3(gamma_k-1)
  xi_k/1 -> Subsystem2/2(xi_k), Subsystem1/2(xi_k)  "xi_k"
  Subsystem1/1(theta_k) -> theta_d_k/1
  reset/1 -> Subsystem2/1(reset), Subsystem1/1(reset)
  Demux/2 -> Subsystem2/4(psi_k)
  psi_k/1 -> Demux/1  "psi_k"
  Demux/1 -> Subsystem1/4(psi_k)
  Subsystem2/1(theta_k) -> theta_q_k1/1

== system Reforce_Experiment_FCS/Control_Scheme/DQ_DTC/Identification_and_Safeguard/Brosch RLS/i_d_RLS/Subsystem ==
  xi_k : Inport
  P_k-1 : Inport  Port=2
  lambda : Inport  Port=3
  Product : Product  Inputs=3  Multiplication=Matrix(*)
  Product1 : Product  Inputs=*/
  Product2 : Product  Multiplication=Matrix(*)
  Sum : Sum  Inputs=|++
  Transpose : Math  Operator=transpose  SaturateOnIntegerOverflow=on
  gamma_k-1 : Outport
  wires:
  Product1/1 -> gamma_k-1/1  "gamma_k-1"
  Product2/1 -> Product1/1
  xi_k/1 -> Product2/2, Product/3, Transpose/1
  Sum/1 -> Product1/2
  P_k-1/1 -> Product/2, Product2/1
  lambda/1 -> Sum/2
  Transpose/1 -> Product/1
  Product/1 -> Sum/1

== system Reforce_Experiment_FCS/Control_Scheme/DQ_DTC/Identification_and_Safeguard/Brosch RLS/i_d_RLS/Subsystem2 ==
  reset : Inport
  xi_k : Inport  Port=2
  gamma_k-1 : Inport  Port=3
  lambda : Inport  Port=4
  Add1 : Sum  Inputs=+-
  Constant2 : Constant  Value=eye(controller.RLS.n)
  Delay : Delay  DelayLength=1  InitialCondition=controller.RLS.P_0  ExternalReset=Rising
      settings: InputPortMap=u0,r5
  Product5 : Product  Multiplication=Matrix(*)
  Product6 : Product  Inputs=*/
  Product7 : Product  Multiplication=Matrix(*)
  Transpose : Math  Operator=transpose  SaturateOnIntegerOverflow=on
  P_k-1 : Outport
  wires:
  Constant2/1 -> Add1/1
  gamma_k-1/1 -> Product7/1
  Delay/1 -> P_k-1/1, Product5/2  "P_k-1"
  Product6/1 -> Product5/1
  xi_k/1 -> Transpose/1
  Product7/1 -> Add1/2  "P_k"
  Add1/1 -> Product6/1
  lambda/1 -> Product6/2
  Product5/1 -> Delay/1  "P_k"
  Transpose/1 -> Product7/2
  reset/1 -> Delay/2

== system Reforce_Experiment_FCS/Control_Scheme/DQ_DTC/Identification_and_Safeguard/Horizon1Predictor/For Each Subsystem/Predictor1 ==
  Ai_plus_E : Inport
  I_minus_A : Inport  Port=2
  B : Inport  Port=3
  B_inv : Inport  Port=4
  E : Inport  Port=5
  u_dq : Inport  Port=6
  Add : Sum  Inputs=2
  Add1 : Sum  Inputs=+-
  Matrix Multiply1 : Product  Multiplication=Matrix(*)
  Matrix Multiply2 : Product  Multiplication=Matrix(*)
  Matrix Multiply3 : Product  Multiplication=Matrix(*)
  i_dq[k+2] : Outport
  u_dq[k+2] : Outport  Port=2
  wires:
  Matrix Multiply1/1 -> Add/2
  u_dq/1 -> Matrix Multiply1/2
  B/1 -> Matrix Multiply1/1
  Add/1 -> Matrix Multiply2/2, i_dq[k+2]/1
  Add1/1 -> Matrix Multiply3/2
  B_inv/1 -> Matrix Multiply3/1
  Matrix Multiply3/1 -> u_dq[k+2]/1
  Ai_plus_E/1 -> Add/1
  I_minus_A/1 -> Matrix Multiply2/1
  Matrix Multiply2/1 -> Add1/1
  E/1 -> Add1/2

== system Reforce_Experiment_FCS/Control_Scheme/DQ_DTC/Identification_and_Safeguard/Horizon1Predictor/For Each Subsystem/VoltageApplier1 ==
  nextControlSignal : Inport
  lastControlSignal : Inport  Port=2
  u_DC : Inport  Port=3
  i_abc : Inport  Port=4
  epsilon : Inport  Port=5
  T_interlock : Inport  Port=6
  i_threshold : Inport  Port=7
  Constant1 : Constant  Value=Ts
  Constant2 : Constant  Value=[0 0 0]
  Constant3 : Constant  Value=controller.compensate_deadtime
  Divide : Product  Inputs=**
  Gain2 : Gain  Gain=1 / 2
  Multiport Switch4 : MultiPortSwitch  DataPortOrder=Specify indices  DataPortIndices={0,1}  DataPortForDefault=Additional data port
  VoltageCorrection : Subsystem
  abc2dq1 : Subsystem
  u_dq[k+1] : Outport
  wires:
  epsilon/1 -> abc2dq1/2(epsilon)
  abc2dq1/1(dq) -> u_dq[k+1]/1
  nextControlSignal/1 -> Divide/2, VoltageCorrection/2(nextControlSignal)
  u_DC/1 -> Gain2/1
  Constant1/1 -> VoltageCorrection/7(T_S)
  T_interlock/1 -> VoltageCorrection/6(T_Interlock)
  i_threshold/1 -> VoltageCorrection/5(i_Threshold)
  Divide/1 -> Multiport Switch4/2
  VoltageCorrection/1(u_abc) -> Multiport Switch4/3
  Multiport Switch4/1 -> abc2dq1/1(abc)
  Constant2/1 -> Multiport Switch4/4
  i_abc/1 -> VoltageCorrection/4(i_abc)
  Gain2/1 -> VoltageCorrection/1(u_DC/2), Divide/1
  lastControlSignal/1 -> VoltageCorrection/3(lastControlSignal)
  Constant3/1 -> Multiport Switch4/1

== system Reforce_Experiment_FCS/Control_Scheme/DQ_DTC/Identification_and_Safeguard/Brosch RLS/i_d_RLS/RLS/Subsystem1 ==
  reset : Inport
  xi_k : Inport  Port=2
  gamma_k-1 : Inport  Port=3
  psi_k : Inport  Port=4
  Add : Sum  Inputs=+-
  Delay1 : Delay  DelayLength=1  InitialCondition=controller.RLS.theta_0  ExternalReset=Rising
      settings: InputPortMap=u0,r5
  Product3 : Product
  Product4 : Product  Multiplication=Matrix(*)
  Sum1 : Sum  Inputs=|++
  Transpose : Math  Operator=transpose  SaturateOnIntegerOverflow=on
  theta_k : Outport
  wires:
  Delay1/1 -> Sum1/1, Product4/2  "theta_k-1"
  Product3/1 -> Sum1/2
  Product4/1 -> Add/2
  Sum1/1 -> theta_k/1, Delay1/1  "theta_k"
  Add/1 -> Product3/2
  psi_k/1 -> Add/1
  gamma_k-1/1 -> Product3/1
  Transpose/1 -> Product4/1
  xi_k/1 -> Transpose/1
  reset/1 -> Delay1/2

== system Reforce_Experiment_FCS/Control_Scheme/DQ_DTC/Identification_and_Safeguard/Brosch RLS/i_d_RLS/RLS/Subsystem2 ==
  reset : Inport
  xi_k : Inport  Port=2
  gamma_k-1 : Inport  Port=3
  psi_k : Inport  Port=4
  Add : Sum  Inputs=+-
  Delay1 : Delay  DelayLength=1  InitialCondition=controller.RLS.theta_0  ExternalReset=Rising
      settings: InputPortMap=u0,r5
  Product3 : Product
  Product4 : Product  Multiplication=Matrix(*)
  Sum1 : Sum  Inputs=|++
  Transpose : Math  Operator=transpose  SaturateOnIntegerOverflow=on
  theta_k : Outport
  wires:
  Delay1/1 -> Sum1/1, Product4/2  "theta_k-1"
  Product3/1 -> Sum1/2
  Product4/1 -> Add/2
  Sum1/1 -> theta_k/1, Delay1/1  "theta_k"
  Add/1 -> Product3/2
  psi_k/1 -> Add/1
  gamma_k-1/1 -> Product3/1
  Transpose/1 -> Product4/1
  xi_k/1 -> Transpose/1
  reset/1 -> Delay1/2

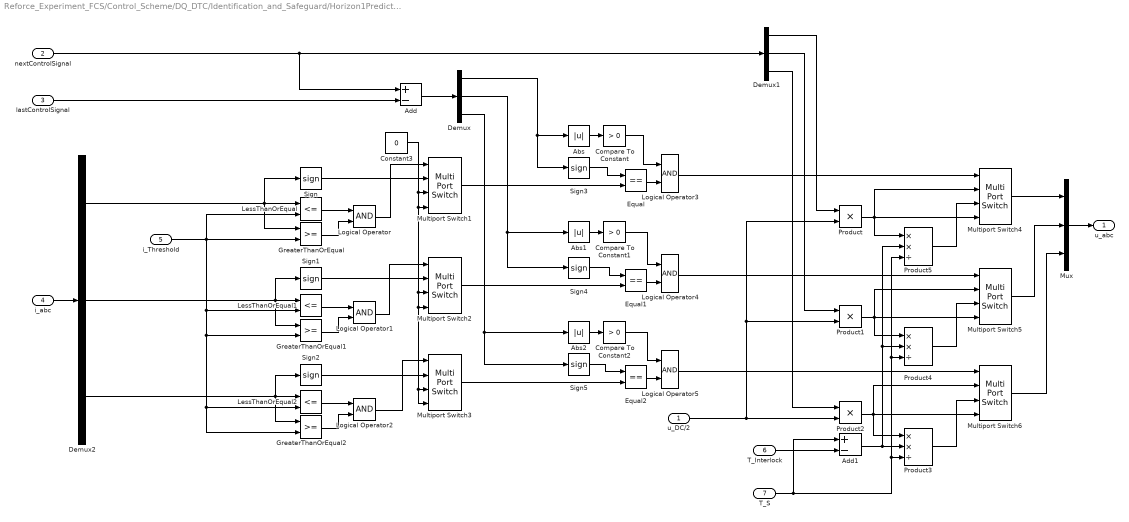
== system Reforce_Experiment_FCS/Control_Scheme/DQ_DTC/Identification_and_Safeguard/Horizon1Predictor/For Each Subsystem/VoltageApplier1/VoltageCorrection ==
  u_DC/2 : Inport
  nextControlSignal : Inport  Port=2
  lastControlSignal : Inport  Port=3
  i_abc : Inport  Port=4
  i_Threshold : Inport  Port=5
  T_Interlock : Inport  Port=6
  T_S : Inport  Port=7
  Abs : Abs
  Abs1 : Abs
  Abs2 : Abs
  Add : Sum  Inputs=+-
  Add1 : Sum  Inputs=+-
  Compare To Constant : simulink/Logic and Bit Operations/Compare To Constant  relop=>  const=0  OutDataTypeStr=boolean
  Compare To Constant1 : simulink/Logic and Bit Operations/Compare To Constant  relop=>  const=0  OutDataTypeStr=boolean
  Compare To Constant2 : simulink/Logic and Bit Operations/Compare To Constant  relop=>  const=0  OutDataTypeStr=boolean
  Constant3 : Constant  Value=0
  Demux : Demux  Outputs=3
  Demux1 : Demux  Outputs=3
  Demux2 : Demux  Outputs=3
  Equal : RelationalOperator  Operator===  OutDataTypeStr=boolean  RndMeth=Simplest
  Equal1 : RelationalOperator  Operator===  OutDataTypeStr=boolean  RndMeth=Simplest
  Equal2 : RelationalOperator  Operator===  OutDataTypeStr=boolean  RndMeth=Simplest
  GreaterThanOrEqual : RelationalOperator  OutDataTypeStr=boolean  RndMeth=Simplest
  GreaterThanOrEqual1 : RelationalOperator  OutDataTypeStr=boolean  RndMeth=Simplest
  GreaterThanOrEqual2 : RelationalOperator  OutDataTypeStr=boolean  RndMeth=Simplest
  LessThanOrEqual : RelationalOperator  Operator=<=  OutDataTypeStr=boolean  RndMeth=Simplest
  LessThanOrEqual1 : RelationalOperator  Operator=<=  OutDataTypeStr=boolean  RndMeth=Simplest
  LessThanOrEqual2 : RelationalOperator  Operator=<=  OutDataTypeStr=boolean  RndMeth=Simplest
  Logical Operator{,1..5} (6 alike) : Logic  AllPortsSameDT=off  OutDataTypeStr=boolean
  Multiport Switch{1..6} (6 alike) : MultiPortSwitch  DataPortOrder=Specify indices  DataPortIndices={0,1}  DataPortForDefault=Additional data port
  Mux : Mux  Inputs=3
  Product : Product
  Product1 : Product
  Product2 : Product
  Product3 : Product  Inputs=**/
  Product4 : Product  Inputs=**/
  Product5 : Product  Inputs=**/
  Sign{,1..5} (6 alike) : Signum
  u_abc : Outport
  wires:
  GreaterThanOrEqual2/1 -> Logical Operator2/2
  Constant3/1 -> Multiport Switch3/4, Multiport Switch3/3, Multiport Switch2/4, Multiport Switch2/3, Multiport Switch1/4, Multiport Switch1/3
  Demux2/1 -> GreaterThanOrEqual/1, Sign/1, LessThanOrEqual/1
  u_DC/2/1 -> Product/2, Product1/2, Product2/2
  T_S/1 -> Product5/3, Product4/3, Product3/3, Add1/1
  Demux/1 -> Sign3/1, Abs/1
  GreaterThanOrEqual1/1 -> Logical Operator1/2
  LessThanOrEqual/1 -> Logical Operator/1
  Add/1 -> Demux/1
  LessThanOrEqual1/1 -> Logical Operator1/1
  Abs2/1 -> Compare To Constant2/1
  Abs/1 -> Compare To Constant/1
  i_Threshold/1 -> LessThanOrEqual/2, GreaterThanOrEqual2/2, LessThanOrEqual2/2, GreaterThanOrEqual1/2, LessThanOrEqual1/2, GreaterThanOrEqual/2
  Product/1 -> Product5/1, Multiport Switch4/4, Multiport Switch4/2
  Add1/1 -> Product4/2, Product5/2, Product3/2
  Abs1/1 -> Compare To Constant1/1
  Multiport Switch6/1 -> Mux/3
  Demux1/2 -> Product1/1
  Multiport Switch1/1 -> Equal/2
  Multiport Switch5/1 -> Mux/2
  Product4/1 -> Multiport Switch5/3
  T_Interlock/1 -> Add1/2
  Logical Operator1/1 -> Multiport Switch2/1
  Logical Operator/1 -> Multiport Switch1/1
  GreaterThanOrEqual/1 -> Logical Operator/2
  nextControlSignal/1 -> Add/1, Demux1/1
  Compare To Constant1/1 -> Logical Operator4/1
  Demux1/1 -> Product/1
  Demux1/3 -> Product2/1
  Logical Operator4/1 -> Multiport Switch5/1
  Product5/1 -> Multiport Switch4/3
  Product1/1 -> Product4/1, Multiport Switch5/4, Multiport Switch5/2
  Logical Operator2/1 -> Multiport Switch3/1
  lastControlSignal/1 -> Add/2
  Compare To Constant/1 -> Logical Operator3/1
  Product2/1 -> Product3/1, Multiport Switch6/4, Multiport Switch6/2
  LessThanOrEqual2/1 -> Logical Operator2/1
  Sign/1 -> Multiport Switch1/2
  Product3/1 -> Multiport Switch6/3
  Logical Operator3/1 -> Multiport Switch4/1
  Sign1/1 -> Multiport Switch2/2
  Sign2/1 -> Multiport Switch3/2
  Logical Operator5/1 -> Multiport Switch6/1
  Compare To Constant2/1 -> Logical Operator5/1
  Multiport Switch4/1 -> Mux/1
  Demux2/2 -> Sign1/1, GreaterThanOrEqual1/1, LessThanOrEqual1/1
  Demux2/3 -> Sign2/1, GreaterThanOrEqual2/1, LessThanOrEqual2/1
  Equal/1 -> Logical Operator3/2
  Sign3/1 -> Equal/1
  Sign4/1 -> Equal1/1
  Multiport Switch2/1 -> Equal1/2
  Demux/2 -> Abs1/1, Sign4/1
  Equal1/1 -> Logical Operator4/2
  Demux/3 -> Sign5/1, Abs2/1
  Multiport Switch3/1 -> Equal2/2
  Sign5/1 -> Equal2/1
  Equal2/1 -> Logical Operator5/2
  Mux/1 -> u_abc/1
  i_abc/1 -> Demux2/1

== system Reforce_Experiment_FCS/Control_Scheme/DQ_DTC/Identification_and_Safeguard/Horizon1Predictor/For Each Subsystem/VoltageApplier1/abc2dq1 ==
  abc : Inport
  epsilon : Inport  Port=2
  Gain1 : Gain  Gain=abc2alphabeta0  Multiplication=Matrix(K*u)
  alphabeta02dq : Subsystem
  dq : Outport
  wires:
  alphabeta02dq/1(dq) -> dq/1
  abc/1 -> Gain1/1
  Gain1/1 -> alphabeta02dq/1(alphabeta0)
  epsilon/1 -> alphabeta02dq/2(epsilon)

== system Reforce_Experiment_FCS/Control_Scheme/DQ_DTC/Identification_and_Safeguard/Horizon1Predictor/For Each Subsystem/VoltageApplier1/abc2dq1/alphabeta02dq ==
  alphabeta0 : Inport
  epsilon : Inport  Port=2
  Cos : Trigonometry  Operator=cos  NumberOfDataPoints=64
  Demux : Demux  Outputs=3
  Gain1 : Gain  Gain=-1
  Gain2 : Gain  Gain=-1
  Mux : Mux  Inputs=2
  Product{,1..3} (4 alike) : Product
  Sin : Trigonometry  NumberOfDataPoints=64
  Sum : Sum  Inputs=|++
  Sum1 : Sum  Inputs=|++
  Terminator : Terminator
  dq : Outport
  wires:
  Gain2/1 -> Cos/1, Sin/1
  Product3/1 -> Sum1/2
  Sin/1 -> Product2/2, Gain1/1
  Product2/1 -> Sum1/1
  Product/1 -> Sum/2
  Gain1/1 -> Product/2
  Demux/2 -> Product/1, Product3/1
  Product1/1 -> Sum/1
  Cos/1 -> Product3/2, Product1/2
  Demux/1 -> Product2/1, Product1/1
  Mux/1 -> dq/1
  Sum1/1 -> Mux/2
  Sum/1 -> Mux/1
  Demux/3 -> Terminator/1
  alphabeta0/1 -> Demux/1
  epsilon/1 -> Gain2/1

== matlab function Reforce_Experiment_FCS/Control_Scheme/DQ_DTC/Action_Processing/EpsilonSafetyActionSelection_old ==
  settings: updateMethod=DISCRETE
  data: argmax_Q input; a_out output int32; a_policy output; a_allowed input; a_current input; epsilon input; safeguard_active output; controller parameter
function [a_out, a_policy, safeguard_active]= fcn(argmax_Q, a_allowed, a_current, epsilon, controller)

a_allowed = a_allowed(~isnan(a_allowed));
safeguard_active = 1;

if rand < epsilon
    % determine action from momentary policy
    a_policy = int32(randi(controller.DQDTC.action_dim))-1;
else
    a_policy = argmax_Q;
end

if isempty(a_allowed)
    % if no action can comply with the op.limits, 
    % apply action that minimizes current
    [~, I] = min(a_current); % argmin
    a_out = int32(I-1);
else
    if ismember(a_policy, a_allowed)
        % apply action that is optimal according to DQN
        a_out = a_policy;  
        safeguard_active = 0;
    else
        % if policy action does not comply with op.limits, apply random
        % action that does
        random_index = randi(length(a_allowed));
        a_out = int32(a_allowed(random_index));
    end
end

== matlab function Reforce_Experiment_FCS/Control_Scheme/DQ_DTC/Learning_Rate_Schedule ==
  data: time input; lr output; controller parameter; epsilon output
function [lr, epsilon] = fcn(time, controller)

alpha = time / controller.DQDTC.schedule_time;

lr = (1-alpha) * controller.DQDTC.initial_lr + alpha * controller.DQDTC.final_lr;
epsilon = (1-alpha) * controller.DQDTC.initial_epsilon + alpha * controller.DQDTC.final_epsilon;

if time >= controller.DQDTC.schedule_time
    lr = controller.DQDTC.final_lr;
    epsilon = controller.DQDTC.final_epsilon;
end

== matlab function Reforce_Experiment_FCS/Control_Scheme/MATLAB Function1 ==
  data: HotButton input; y output; schedulerClock input; stop input
function y = fcn(HotButton, schedulerClock, stop)
persistent learning block_start
if isempty(learning)
    learning = false;
    block_start = false;
end

if HotButton && not((schedulerClock == 0.0) || stop) && not(block_start)
    learning = true;
elseif (schedulerClock == 0.0) || stop
    learning = false;
    block_start = true;
end

if not(stop) && not(HotButton)
    block_start = false;
end

y = learning;

== stateflow chart Reforce_Experiment_FCS/Control_Scheme/Chart ==
  state Waiting
    entry:
    idx = 0;
    T_out = 0;
    exit:
    idx = idx + 1;
  state Active
    entry:
    T_out = T_ref(idx);
    exit:
    idx = idx + 1;
  (default) -> Waiting
  (junction 14) -> Waiting [order 1] : [idx >= length(T_ref)]
  Waiting -> Active : [activate]
  Active -> (junction 14) : [after(0.5, sec)]
  (junction 14) -> Active [order 2]
  data: activate input; T_out output; idx local; T_ref parameter

== matlab function Reforce_Experiment_FCS/Control_Scheme/DQ_DTC/Action_Processing/EpsilonSafetyActionSelection ==
  settings: updateMethod=DISCRETE
  data: Q_values input; a_out output int32; a_policy output; a_allowed input; a_current input; epsilon input; safeguard_active output
function [a_out, a_policy, safeguard_active]= fcn(Q_values, a_allowed, a_current, epsilon)

a_allowed = a_allowed(~isnan(a_allowed));
safeguard_active = 1;

if rand < epsilon
    % determine action from momentary policy
    a_policy = int32(randi(length(Q_values))-1);

    if ismember(a_policy, a_allowed)
        a_out = a_policy;
        safeguard_active = 0;
    else
        if isempty(a_allowed)
            [~, I] = min(a_current); % argmin
            a_out = int32(I-1);
        else
            random_index = randi(length(a_allowed));    
            a_out = int32(a_allowed(random_index));
        end
    end

else
    [~, I] = max(Q_values);
    a_policy = int32(I-1);

    if ismember(a_policy, a_allowed)
        a_out = a_policy;
        safeguard_active = 0;
    else
        if isempty(a_allowed)
            [~, I] = min(a_current); % argmin
            a_out = int32(I-1);
        else
            [~, I] = max(Q_values(a_allowed+1));
            a_out = int32(a_allowed(I));
        end
    end       
end

== matlab function Reforce_Experiment_FCS/Control_Scheme/MATLAB Function ==
  data: u_DC input; chop output; chop_low input; chop_high input; chop_last input
function chop = fcn(u_DC, chop_low, chop_high, chop_last)

%% for PWM chopping

chop = (u_DC - chop_low) / (chop_high - chop_low);

if chop > 1.0
    chop = 1.0;
end

if chop < 0.0
    chop = 0.0;
end


%% for non-PWM chopping
% if u_DC > chop_high
%     chop = true;
% elseif u_DC < chop_low
%     chop = false;
% else
%     chop = chop_last;
end

== matlab function Reforce_Experiment_FCS/Control_Scheme/DQ_DTC/Identification_and_Safeguard/ABE_d_LUT ==
  data: w_me input; A_d output; i_dq input; B_d output; E_d output; controller parameter; motor parameter; Ts parameter
function [A_d, B_d, E_d] = fcn(w_me, i_dq, controller, motor, Ts)

L_dd = LUT2D(controller.preindl.LUT.x_vec,controller.preindl.LUT.y_vec,controller.preindl.LUT.L_dd_map,i_dq(1),i_dq(2));
L_qq = LUT2D(controller.preindl.LUT.x_vec,controller.preindl.LUT.y_vec,controller.preindl.LUT.L_qq_map,i_dq(1),i_dq(2));
L_dq = LUT2D(controller.preindl.LUT.x_vec,controller.preindl.LUT.y_vec,controller.preindl.LUT.L_dq_map,i_dq(1),i_dq(2));
L_qd = LUT2D(controller.preindl.LUT.x_vec,controller.preindl.LUT.y_vec,controller.preindl.LUT.L_qd_map,i_dq(1),i_dq(2));

Psi_d = LUT2D(controller.preindl.LUT.x_vec,controller.preindl.LUT.y_vec,controller.preindl.LUT.Psi_d_map,i_dq(1),i_dq(2));
Psi_q = LUT2D(controller.preindl.LUT.x_vec,controller.preindl.LUT.y_vec,controller.preindl.LUT.Psi_q_map,i_dq(1),i_dq(2)); 


w_el = motor.param.p * w_me;
inv_L = 1 / (L_dd * L_qq - L_dq * L_qd) * [L_qq -L_dq;
                                          -L_qd  L_dd];


A_d = eye(2) - Ts * inv_L * motor.param.R_s;

B_d = Ts * inv_L;

E_d = - Ts * w_el * inv_L * [-Psi_q;
                              Psi_d;];
